simulink model "MTL"  (R2013a)
settings: Solver=ode45  StartTime=0.0  StopTime=1  RelTol=1e-3
libraries: powerlib x34
settings Model: Creator=Sony  LastModifiedBy=Sony

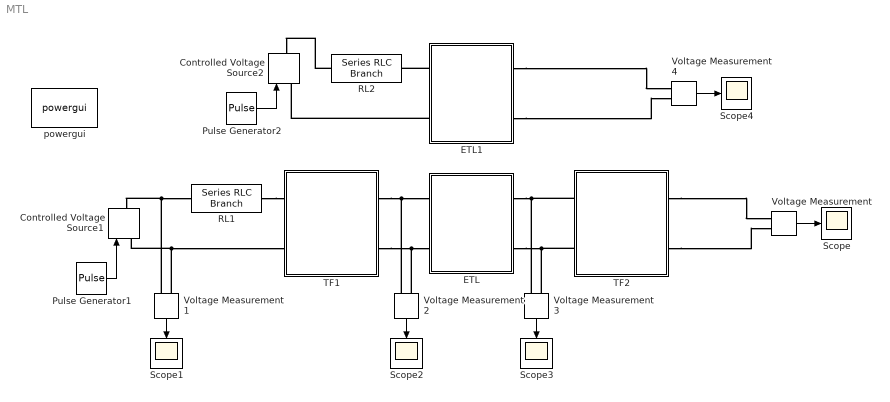
== system MTL ==
  Controlled Voltage Source1 : powerlib/Electrical Sources/Controlled Voltage Source  Initialize=on  Source_Type=AC  Amplitude=0  Phase=0  Frequency=0  Measurements=None
  Controlled Voltage Source2 : powerlib/Electrical Sources/Controlled Voltage Source  Initialize=on  Source_Type=AC  Amplitude=0  Phase=0  Frequency=0  Measurements=None
  ETL : Subsystem
  ETL1 : Subsystem
  Pulse Generator1 : DiscretePulseGenerator  PulseType=Time based  Amplitude=220*sqrt(2)  Period=1/50  PulseWidth=50
  Pulse Generator2 : DiscretePulseGenerator  PulseType=Time based  Amplitude=220*sqrt(2)  Period=1/50  PulseWidth=50
  RL1 : powerlib/Elements/Series RLC Branch  LConnTagsString=__new0  RConnTagsString=__new0  BranchType=R  Resistance=10  Inductance=1e-5  SetiL0=off  InitialCurrent=0  Capacitance=1e-6  Setx0=off  InitialVoltage=0  Measurements=None
  RL2 : powerlib/Elements/Series RLC Branch  LConnTagsString=__new0  RConnTagsString=__new0  BranchType=R  Resistance=10  Inductance=1e-5  SetiL0=off  InitialCurrent=0  Capacitance=1e-6  Setx0=off  InitialVoltage=0  Measurements=None
  Scope{,1..4} (5 alike) : Scope
      Scope settings: YMin=115000  YMax=210000
      Scope1 settings: YMin=0  YMax=325  SaveName=ScopeData2
      Scope2 settings: YMin=0  YMax=400
      Scope3 settings: YMin=125  YMax=205  SaveName=ScopeData3
      Scope4 settings: YMin=-1000  YMax=1300  SaveName=ScopeData4
  TF1 : Subsystem
  TF2 : Subsystem
  Voltage Measurement{,1..4} (5 alike) : powerlib/Measurements/Voltage Measurement  PhasorSimulation=off  OutputType=Complex  PSBequivalent=0
  powergui : powerlib/powergui  Priority=1  SimulationMode=Discrete  SolverType=Tustin  SampleTime=1e-6  frequency=60  SPID=off  DisableSnubberDevices=off  DisableRonSwitches=off  DisableVfSwitches=off  SwTol=0  Interpol=off  DisplayEquations=off  frequencyindice=0  Pbase=100e6  ErrMax=1e-4  Iterations=50  UnitsV=kV  UnitsW=MW  FunctionMessages=off  echomessages=off  HookPort=off  EnableUseOfTLC=off  x0status=blocks  RestoreLinks=warning  ResistiveCurrentMeasurement=off  Frange=[0:2:500]  Ylog=off  Xlog=on  ShowGrid=off  save=off  variable=ZData  ZoomFFT=off  StartTime=0.0  cycles=1  DisplayStyle=1  fundamental=60  FreqAxis=off  MaxFrequency=1000  frequencyindicesteady=1  RmsSteady=1  display=off  Ts=0  methode=off
  wires:
  Voltage Measurement/1 -> Scope/1
  Voltage Measurement1/1 -> Scope1/1
  Pulse Generator1/1 -> Controlled Voltage Source1/1
  Voltage Measurement2/1 -> Scope2/1
  Voltage Measurement3/1 -> Scope3/1
  Pulse Generator2/1 -> Controlled Voltage Source2/1
  Voltage Measurement4/1 -> Scope4/1
  connections:
  TF2/RConn1 -- Voltage Measurement/LConn1
  TF2/RConn2 -- Voltage Measurement/LConn2
  ETL/RConn1 -- TF2/LConn1 -- Voltage Measurement3/LConn1
  ETL/RConn2 -- TF2/LConn2 -- Voltage Measurement3/LConn2
  TF1/RConn1 -- Voltage Measurement2/LConn1 -- ETL/LConn1
  TF1/RConn2 -- Voltage Measurement2/LConn2 -- ETL/LConn2
  Voltage Measurement1/LConn2 -- TF1/LConn2 -- Controlled Voltage Source1/LConn1
  Voltage Measurement1/LConn1 -- RL1/LConn1 -- Controlled Voltage Source1/RConn1
  RL1/RConn1 -- TF1/LConn1
  ETL1/LConn2 -- Controlled Voltage Source2/LConn1
  RL2/LConn1 -- Controlled Voltage Source2/RConn1
  ETL1/RConn1 -- Voltage Measurement4/LConn1
  ETL1/RConn2 -- Voltage Measurement4/LConn2
  ETL1/LConn1 -- RL2/RConn1

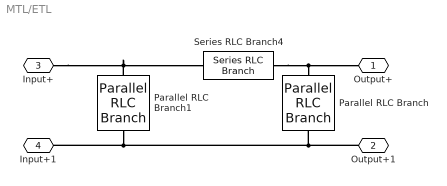
== system MTL/ETL ==
  Parallel RLC Branch : powerlib/Elements/Parallel RLC Branch  LConnTagsString=a  RConnTagsString=__new0  BranchType=C  Resistance=1  Inductance=1e-3  SetiL0=off  InitialCurrent=0  Capacitance=4e-6  Setx0=off  InitialVoltage=0  Measurements=None
  Parallel RLC Branch1 : powerlib/Elements/Parallel RLC Branch  LConnTagsString=a  RConnTagsString=__new0  BranchType=C  Resistance=1  Inductance=1e-3  SetiL0=off  InitialCurrent=0  Capacitance=4e-6  Setx0=off  InitialVoltage=0  Measurements=None
  Series RLC Branch4 : powerlib/Elements/Series RLC Branch  LConnTagsString=__new0  RConnTagsString=__new0  BranchType=RL  Resistance=4  Inductance=0.3  SetiL0=off  InitialCurrent=0  Capacitance=1e-6  Setx0=off  InitialVoltage=0  Measurements=None
  Output+ : PMIOPort  Port=1  Side=Right
  Output+1 : PMIOPort  Port=2  Side=Right
  Input+ : PMIOPort  Port=3  Side=Left
  Input+1 : PMIOPort  Port=4  Side=Left
  connections:
  Output+1/RConn1 -- Parallel RLC Branch1/RConn1 -- Input+1/RConn1 -- Parallel RLC Branch/RConn1
  Input+/RConn1 -- Parallel RLC Branch1/LConn1 -- Series RLC Branch4/LConn1
  Series RLC Branch4/RConn1 -- Output+/RConn1 -- Parallel RLC Branch/LConn1

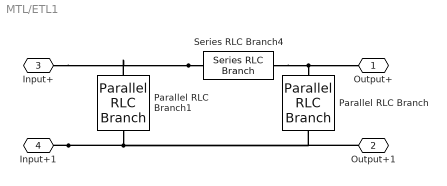
== system MTL/ETL1 ==
  Parallel RLC Branch : powerlib/Elements/Parallel RLC Branch  LConnTagsString=a  RConnTagsString=__new0  BranchType=C  Resistance=1  Inductance=1e-3  SetiL0=off  InitialCurrent=0  Capacitance=4e-6  Setx0=off  InitialVoltage=0  Measurements=None
  Parallel RLC Branch1 : powerlib/Elements/Parallel RLC Branch  LConnTagsString=a  RConnTagsString=__new0  BranchType=C  Resistance=1  Inductance=1e-3  SetiL0=off  InitialCurrent=0  Capacitance=4e-6  Setx0=off  InitialVoltage=0  Measurements=None
  Series RLC Branch4 : powerlib/Elements/Series RLC Branch  LConnTagsString=__new0  RConnTagsString=__new0  BranchType=RL  Resistance=4  Inductance=0.3  SetiL0=off  InitialCurrent=0  Capacitance=1e-6  Setx0=off  InitialVoltage=0  Measurements=None
  Output+ : PMIOPort  Port=1  Side=Right
  Output+1 : PMIOPort  Port=2  Side=Right
  Input+ : PMIOPort  Port=3  Side=Left
  Input+1 : PMIOPort  Port=4  Side=Left
  connections:
  Input+1/RConn1 -- Output+1/RConn1 -- Parallel RLC Branch/RConn1 -- Parallel RLC Branch1/RConn1
  Series RLC Branch4/LConn1 -- Input+/RConn1 -- Parallel RLC Branch1/LConn1
  Series RLC Branch4/RConn1 -- Parallel RLC Branch/LConn1 -- Output+/RConn1

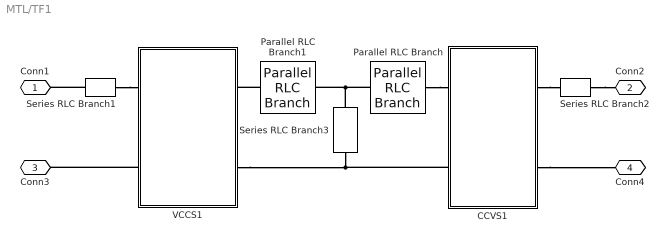
== system MTL/TF1 ==
  CCVS1 : Subsystem  mask{N=1000}
  Parallel RLC Branch : powerlib/Elements/Parallel RLC Branch  LConnTagsString=a  RConnTagsString=__new0  BranchType=RL  Resistance=1e4  Inductance=1e-4  SetiL0=off  InitialCurrent=0  Capacitance=1e-6  Setx0=off  InitialVoltage=0  Measurements=None
  Parallel RLC Branch1 : powerlib/Elements/Parallel RLC Branch  LConnTagsString=a  RConnTagsString=__new0  BranchType=RL  Resistance=1e4  Inductance=1e-4  SetiL0=off  InitialCurrent=0  Capacitance=1e-6  Setx0=off  InitialVoltage=0  Measurements=None
  Series RLC Branch1 : powerlib/Elements/Series RLC Branch  LConnTagsString=__new0  RConnTagsString=__new0  BranchType=RL  Resistance=.1  Inductance=1e-5  SetiL0=off  InitialCurrent=0  Capacitance=1e-6  Setx0=off  InitialVoltage=0  Measurements=None
  Series RLC Branch2 : powerlib/Elements/Series RLC Branch  LConnTagsString=__new0  RConnTagsString=__new0  BranchType=RL  Resistance=.1  Inductance=1e-5  SetiL0=off  InitialCurrent=0  Capacitance=1e-6  Setx0=off  InitialVoltage=0  Measurements=None
  Series RLC Branch3 : powerlib/Elements/Series RLC Branch  LConnTagsString=__new0  RConnTagsString=__new0  BranchType=C  Resistance=1  Inductance=1e-3  SetiL0=off  InitialCurrent=0  Capacitance=1e9  Setx0=off  InitialVoltage=0  Measurements=None
  VCCS1 : Subsystem  mask{N=100}
  Conn1 : PMIOPort  Port=1  Side=Left
  Conn2 : PMIOPort  Port=2  Side=Right
  Conn3 : PMIOPort  Port=3  Side=Left
  Conn4 : PMIOPort  Port=4  Side=Right
  connections:
  Series RLC Branch1/LConn1 -- Conn1/RConn1
  CCVS1/RConn1 -- Series RLC Branch2/LConn1
  CCVS1/RConn2 -- Conn4/RConn1
  VCCS1/LConn2 -- Conn3/RConn1
  VCCS1/RConn2 -- CCVS1/LConn2 -- Series RLC Branch3/RConn1
  Parallel RLC Branch/LConn1 -- Parallel RLC Branch1/RConn1 -- Series RLC Branch3/LConn1
  Parallel RLC Branch/RConn1 -- CCVS1/LConn1
  Series RLC Branch1/RConn1 -- VCCS1/LConn1
  Series RLC Branch2/RConn1 -- Conn2/RConn1
  Parallel RLC Branch1/LConn1 -- VCCS1/RConn1

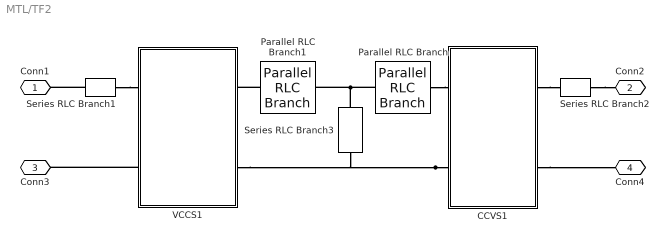
== system MTL/TF2 ==
  CCVS1 : Subsystem  mask{N=100}
  Parallel RLC Branch : powerlib/Elements/Parallel RLC Branch  LConnTagsString=a  RConnTagsString=__new0  BranchType=RL  Resistance=1e4  Inductance=1e-4  SetiL0=off  InitialCurrent=0  Capacitance=1e-6  Setx0=off  InitialVoltage=0  Measurements=None
  Parallel RLC Branch1 : powerlib/Elements/Parallel RLC Branch  LConnTagsString=a  RConnTagsString=__new0  BranchType=RL  Resistance=1e4  Inductance=1e-4  SetiL0=off  InitialCurrent=0  Capacitance=1e-6  Setx0=off  InitialVoltage=0  Measurements=None
  Series RLC Branch1 : powerlib/Elements/Series RLC Branch  LConnTagsString=__new0  RConnTagsString=__new0  BranchType=RL  Resistance=.1  Inductance=1e-5  SetiL0=off  InitialCurrent=0  Capacitance=1e-6  Setx0=off  InitialVoltage=0  Measurements=None
  Series RLC Branch2 : powerlib/Elements/Series RLC Branch  LConnTagsString=__new0  RConnTagsString=__new0  BranchType=RL  Resistance=.1  Inductance=1e-5  SetiL0=off  InitialCurrent=0  Capacitance=1e-6  Setx0=off  InitialVoltage=0  Measurements=None
  Series RLC Branch3 : powerlib/Elements/Series RLC Branch  LConnTagsString=__new0  RConnTagsString=__new0  BranchType=C  Resistance=1  Inductance=1e-3  SetiL0=off  InitialCurrent=0  Capacitance=1e9  Setx0=off  InitialVoltage=0  Measurements=None
  VCCS1 : Subsystem  mask{N=1000}
  Conn1 : PMIOPort  Port=1  Side=Left
  Conn2 : PMIOPort  Port=2  Side=Right
  Conn3 : PMIOPort  Port=3  Side=Left
  Conn4 : PMIOPort  Port=4  Side=Right
  connections:
  Series RLC Branch1/LConn1 -- Conn1/RConn1
  CCVS1/RConn1 -- Series RLC Branch2/LConn1
  CCVS1/RConn2 -- Conn4/RConn1
  VCCS1/LConn2 -- Conn3/RConn1
  CCVS1/LConn2 -- VCCS1/RConn2 -- Series RLC Branch3/RConn1
  Parallel RLC Branch/LConn1 -- Parallel RLC Branch1/RConn1 -- Series RLC Branch3/LConn1
  Parallel RLC Branch/RConn1 -- CCVS1/LConn1
  Series RLC Branch1/RConn1 -- VCCS1/LConn1
  Series RLC Branch2/RConn1 -- Conn2/RConn1
  Parallel RLC Branch1/LConn1 -- VCCS1/RConn1

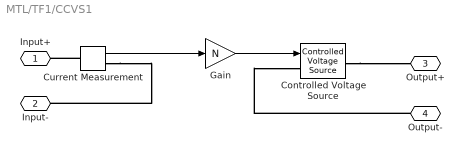
== system MTL/TF1/CCVS1 ==
  Controlled Voltage Source : powerlib/Electrical Sources/Controlled Voltage Source  Initialize=on  Source_Type=AC  Amplitude=0  Phase=0  Frequency=0  Measurements=None
  Current Measurement : powerlib/Measurements/Current Measurement  PhasorSimulation=off  OutputType=Complex  PSBequivalent=0
  Gain : Gain  Gain=N
  Input+ : PMIOPort  Port=1  Side=Left
  Input- : PMIOPort  Port=2  Side=Left
  Output+ : PMIOPort  Port=3  Side=Right
  Output- : PMIOPort  Port=4  Side=Right
  wires:
  Gain/1 -> Controlled Voltage Source/1
  Current Measurement/1 -> Gain/1
  connections:
  Current Measurement/LConn1 -- Input+/RConn1
  Current Measurement/RConn1 -- Input-/RConn1
  Controlled Voltage Source/RConn1 -- Output+/RConn1
  Output-/RConn1 -- Controlled Voltage Source/LConn1

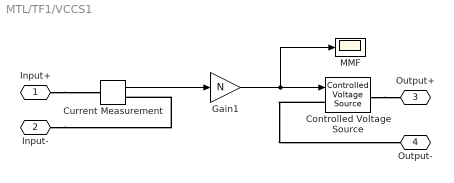
== system MTL/TF1/VCCS1 ==
  Controlled Voltage Source : powerlib/Electrical Sources/Controlled Voltage Source  Initialize=on  Source_Type=AC  Amplitude=0  Phase=0  Frequency=0  Measurements=None
  Current Measurement : powerlib/Measurements/Current Measurement  PhasorSimulation=off  OutputType=Complex  PSBequivalent=0
  Gain1 : Gain  Gain=N
  MMF : Scope
      settings: YMin=-2500  YMax=17500  SaveName=ScopeData8
  Input+ : PMIOPort  Port=1  Side=Left
  Input- : PMIOPort  Port=2  Side=Left
  Output+ : PMIOPort  Port=3  Side=Right
  Output- : PMIOPort  Port=4  Side=Right
  wires:
  Current Measurement/1 -> Gain1/1
  Gain1/1 -> MMF/1, Controlled Voltage Source/1
  connections:
  Input+/RConn1 -- Current Measurement/LConn1
  Input-/RConn1 -- Current Measurement/RConn1
  Controlled Voltage Source/RConn1 -- Output+/RConn1
  Controlled Voltage Source/LConn1 -- Output-/RConn1

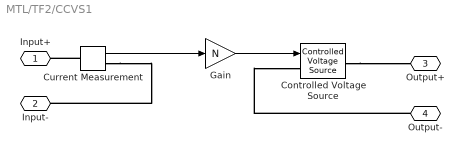
== system MTL/TF2/CCVS1 ==
  Controlled Voltage Source : powerlib/Electrical Sources/Controlled Voltage Source  Initialize=on  Source_Type=AC  Amplitude=0  Phase=0  Frequency=0  Measurements=None
  Current Measurement : powerlib/Measurements/Current Measurement  PhasorSimulation=off  OutputType=Complex  PSBequivalent=0
  Gain : Gain  Gain=N
  Input+ : PMIOPort  Port=1  Side=Left
  Input- : PMIOPort  Port=2  Side=Left
  Output+ : PMIOPort  Port=3  Side=Right
  Output- : PMIOPort  Port=4  Side=Right
  wires:
  Gain/1 -> Controlled Voltage Source/1
  Current Measurement/1 -> Gain/1
  connections:
  Current Measurement/LConn1 -- Input+/RConn1
  Current Measurement/RConn1 -- Input-/RConn1
  Controlled Voltage Source/RConn1 -- Output+/RConn1
  Output-/RConn1 -- Controlled Voltage Source/LConn1

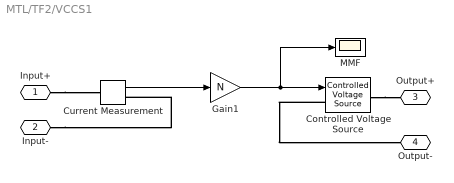
== system MTL/TF2/VCCS1 ==
  Controlled Voltage Source : powerlib/Electrical Sources/Controlled Voltage Source  Initialize=on  Source_Type=AC  Amplitude=0  Phase=0  Frequency=0  Measurements=None
  Current Measurement : powerlib/Measurements/Current Measurement  PhasorSimulation=off  OutputType=Complex  PSBequivalent=0
  Gain1 : Gain  Gain=N
  MMF : Scope
      settings: YMin=-2500  YMax=17500  SaveName=ScopeData8
  Input+ : PMIOPort  Port=1  Side=Left
  Input- : PMIOPort  Port=2  Side=Left
  Output+ : PMIOPort  Port=3  Side=Right
  Output- : PMIOPort  Port=4  Side=Right
  wires:
  Current Measurement/1 -> Gain1/1
  Gain1/1 -> MMF/1, Controlled Voltage Source/1
  connections:
  Input+/RConn1 -- Current Measurement/LConn1
  Input-/RConn1 -- Current Measurement/RConn1
  Controlled Voltage Source/RConn1 -- Output+/RConn1
  Controlled Voltage Source/LConn1 -- Output-/RConn1
